simulink model "diff_mobile_model_simple"  (R2015b)
settings: Solver=ode5  StartTime=0.0  StopTime=inf  FixedStep=0.001  RelTol=1e-3
values from neighbouring files (symbols this model uses):
  Ki_L = (9.11/1)*Kp_L*1    (= 292.65875)    [bode_V.m]
  Kp_L = 25.7/0.8    (= 32.125)    [bode_V.m]
  s = tf('s')    [bode.m]    (also in bode_V.m; bode_delay.m; model_emf_compensation.m; motor_damping_with_step_response.m)
  Ts = 0.02    [ID_freq.m]    (also in bode.m = 0.01; bode_V.m = 0.001; bode_delay.m = 0.04; motor_damping_with_step_response.m = 0.01)
undefined symbols (not defined in the file or in its folder): Ki_W, Kp_W
libraries: cstblocks x6, aerolibanimutils x1
settings Model: Creator=root  LastModifiedBy=root

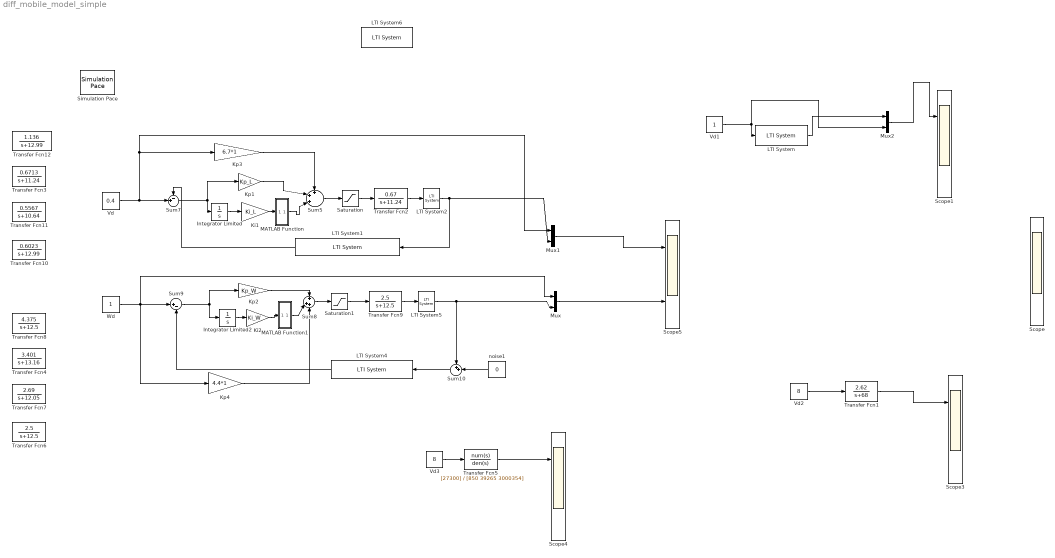
== system diff_mobile_model_simple ==
  Integrator Limited : Integrator  UpperSaturationLimit=24  LowerSaturationLimit=-24
  Integrator Limited2 : Integrator  UpperSaturationLimit=2500  LowerSaturationLimit=-2500
  Ki1 : Gain  Gain=Ki_L
  Ki2 : Gain  Gain=Ki_W
  Kp1 : Gain  Gain=Kp_L
  Kp2 : Gain  Gain=Kp_W
  Kp3 : Gain  Gain=6.7*1
  Kp4 : Gain  Gain=4.4*1
  LTI System : cstblocks/LTI System  sys=tf(1,[0 1],'InputDelay',0.04)  IC=[]
  LTI System1 : cstblocks/LTI System  sys=(1-exp(-Ts*s))/(Ts*s)  IC=[]
  LTI System2 : cstblocks/LTI System  sys=tf(1,[0 1],'InputDelay',0.052)  IC=[]
  LTI System4 : cstblocks/LTI System  sys=(1-exp(-Ts*s))/(Ts*s)  IC=[]
  LTI System5 : cstblocks/LTI System  sys=tf(1,[0 1],'InputDelay',0.052)  IC=[]
  LTI System6 : cstblocks/LTI System  sys=((1-exp(-100*s))/(1-exp(-1*s)))/100  IC=[]
  MATLAB Function : MATLAB Function  TreatAsAtomicUnit=on
  MATLAB Function1 : MATLAB Function  TreatAsAtomicUnit=on
  Mux : Mux  Inputs=2
  Mux1 : Mux  Inputs=2
  Mux2 : Mux  Inputs=2
  Saturation : Saturate  UpperLimit=24  LowerLimit=-24
  Saturation1 : Saturate  UpperLimit=24  LowerLimit=-24
  Scope : Scope  NumInputPorts=4
  Scope{1,3..5} (4 alike) : Scope  NumInputPorts=2
  Simulation Pace : aerolibanimutils/Simulation Pace  SimulationPace=1  SleepMode=MATLAB Thread  OutputPaceError=off  SampleTime=-1
  Sum10 : Sum  Inputs=++|
  Sum5 : Sum  Inputs=+++|
  Sum7 : Sum  Inputs=-+|
  Sum8 : Sum  Inputs=+|++
  Sum9 : Sum  Inputs=|+-
  Transfer Fcn1 : TransferFcn  Numerator=[2.62]  Denominator=[1 68]
  Transfer Fcn10 : TransferFcn  Numerator=[0.6023]  Denominator=[1 12.99]
  Transfer Fcn11 : TransferFcn  Numerator=[0.5567]  Denominator=[1 10.64]
  Transfer Fcn12 : TransferFcn  Numerator=[1.136]  Denominator=[1 12.99]
  Transfer Fcn2 : TransferFcn  Numerator=[0.67]  Denominator=[1 11.24]
  Transfer Fcn3 : TransferFcn  Numerator=[0.6713]  Denominator=[1 11.24]
  Transfer Fcn4 : TransferFcn  Numerator=[3.401]  Denominator=[1 13.16]
  Transfer Fcn5 : TransferFcn  Numerator=[27300]  Denominator=[850 39265 3000354]
  Transfer Fcn6 : TransferFcn  Numerator=[2.5]  Denominator=[1 12.5]
  Transfer Fcn7 : TransferFcn  Numerator=[2.69]  Denominator=[1 12.05]
  Transfer Fcn8 : TransferFcn  Numerator=[4.375]  Denominator=[1 12.5]
  Transfer Fcn9 : TransferFcn  Numerator=[2.5]  Denominator=[1 12.5]
  Vd : Constant  Value=0.4
  Vd1 : Constant
  Vd2 : Constant  Value=8
  Vd3 : Constant  Value=8
  Wd : Constant
  noise1 : Constant  Value=0
  wires:
  Sum7/1 -> Integrator Limited/1, Kp1/1
  Vd/1 -> Sum7/2, Mux1/1, Kp3/1
  Kp2/1 -> Sum8/1
  Ki2/1 -> MATLAB Function1/1(u)
  Sum9/1 -> Integrator Limited2/1, Kp2/1
  Wd/1 -> Sum9/1, Kp4/1, Mux/1
  noise1/1 -> Sum10/2
  Sum10/1 -> LTI System4/1
  Transfer Fcn9/1 -> LTI System5/1
  Transfer Fcn2/1 -> LTI System2/1
  Vd1/1 -> Mux2/2, LTI System/1
  LTI System/1 -> Mux2/1
  Mux2/1 -> Scope1/1
  Sum5/1 -> Saturation/1
  Saturation/1 -> Transfer Fcn2/1
  LTI System2/1 -> LTI System1/1, Mux1/2
  Vd2/1 -> Transfer Fcn1/1
  Transfer Fcn1/1 -> Scope3/1
  Kp3/1 -> Sum5/1
  Kp1/1 -> Sum5/2
  Ki1/1 -> MATLAB Function/1(u)
  Vd3/1 -> Transfer Fcn5/1
  Transfer Fcn5/1 -> Scope4/1
  Mux1/1 -> Scope5/1
  Sum8/1 -> Saturation1/1
  LTI System4/1 -> Sum9/2
  Saturation1/1 -> Transfer Fcn9/1
  LTI System5/1 -> Sum10/1, Mux/2
  Kp4/1 -> Sum8/3
  Mux/1 -> Scope5/2
  Integrator Limited/1 -> Ki1/1
  Integrator Limited2/1 -> Ki2/1
  LTI System1/1 -> Sum7/1
  MATLAB Function/1(y) -> Sum5/3
  MATLAB Function1/1(y) -> Sum8/2

== matlab function diff_mobile_model_simple/MATLAB Function1 ==
  data: u input; y output
function y = fcn(u)
%#codegen

if u >=20
    y=20;
else if u<=-20
        y=-20;
    else
        y=u;
    end
end
end

== matlab function diff_mobile_model_simple/MATLAB Function ==
  data: u input; y output
function y = fcn(u)
%#codegen

if u >=22
    y=22;
else if u<=-22
        y=-22;
    else
        y=u;
    end
end
end
